simulink model "task3"  (R2023a)
settings: Solver=FixedStepAuto  StartTime=0.0  StopTime=10.0  RelTol=1e-3
libraries: simulink x9
settings Model: Creator=user  LastModifiedBy=user
settings OptimizationCC: DefaultParameterBehavior=Inlined  UseDivisionForNetSlopeComputation=on  GainParamInheritBuiltInType=on  UseFloatMulNetSlope=on  InlineInvariantSignals=on  PassReuseOutputArgsAs=Individual arguments  ZeroExternalMemoryAtStartup=off  ZeroInternalMemoryAtStartup=off  NoFixptDivByZeroProtection=on  EfficientFloat2IntCast=on  LifeSpan=1  OptimizeBlockOrder=speed  DifferentSizesBufferReuse=on  EfficientTunableParamExpr=on
settings DebuggingCC: ParameterTunabilityLossMsg=error
settings HardwareCC: ProdLongLongMode=on
settings SFSimCC: MATLABDynamicMemAlloc=off
settings RTWCC: Description=Embedded Coder  SystemTargetFile=ert.tlc  TemplateMakefile=ert_default_tmf
settings CodeAppCC: ForceParamTrailComments=on  IgnoreCustomStorageClasses=off  OperatorAnnotations=on  SimulinkDataObjDesc=on  SFDataObjDesc=on  CustomSymbolStrGlobalVar=rt$N$M  CustomSymbolStrType=$N$M  CustomSymbolStrFcn=$N$M$F  CustomSymbolStrMacro=$N$M  InsertBlockDesc=on
settings ERTTargetCC: TargetLangStandard=C99 (ISO)  GenerateSampleERTMain=on  IncludeMdlTerminateFcn=off  CombineSignalStateStructs=on  SupportComplex=off  SupportContinuousTime=on  InlinedParameterPlacement=NonHierarchical  ERTCustomFileTemplate=example_file_process.tlc  ERTFilePackagingFormat=CompactWithDataFile

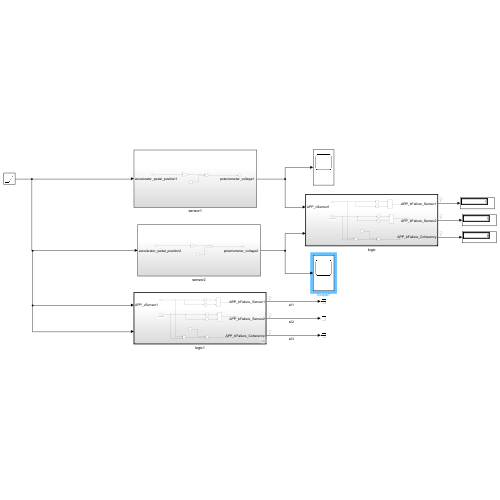
[thumbnail: Simulink's stored preview of the top-level diagram]
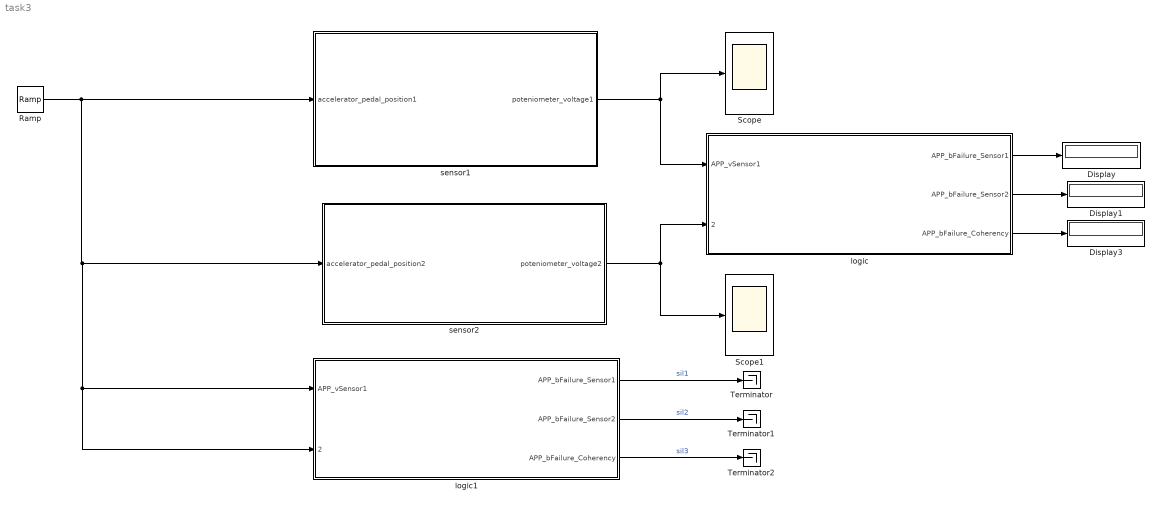
== system task3 ==
  Display : Display
  Display1 : Display
  Display3 : Display
  Ramp : simulink/Sources/Ramp  slope=1  start=0  InitialOutput=0
  Scope : Scope
  Scope1 : Scope
  Terminator : Terminator
  Terminator1 : Terminator
  Terminator2 : Terminator
  logic : Subsystem  TreatAsAtomicUnit=on
  logic1 : Subsystem  TreatAsAtomicUnit=on
  sensor1 : Subsystem
  sensor2 : Subsystem
  wires:
  sensor1/1("poteniometer_voltage1 ") -> Scope/1, logic/1("APP_vSensor1 ")
  sensor2/1("poteniometer_voltage2 ") -> logic/2(" "), Scope1/1
  logic/1(APP_bFailure_Sensor1) -> Display/1
  logic/2(APP_bFailure_Sensor2) -> Display1/1
  logic/3(APP_bFailure_Coherency) -> Display3/1
  Ramp/1 -> logic1/2(" "), logic1/1("APP_vSensor1 "), sensor2/1(accelerator_pedal_position2), sensor1/1("accelerator_pedal_position1 ")
  logic1/1(APP_bFailure_Sensor1) -> Terminator/1  "sil1"
  logic1/2(APP_bFailure_Sensor2) -> Terminator1/1  "sil2"
  logic1/3(APP_bFailure_Coherency) -> Terminator2/1  "sil3"

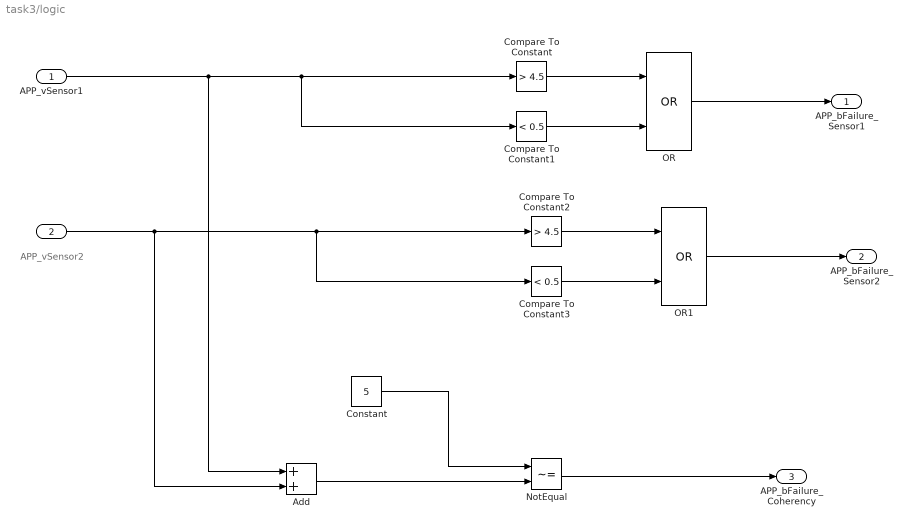
== system task3/logic ==
  note: APP_vSensor2
  "APP_vSensor1 " : Inport
  " " : Inport  Port=2
  Add : Sum
  Compare To Constant : simulink/Logic and Bit Operations/Compare To Constant  relop=>  const=4.5  OutDataTypeStr=boolean
  Compare To Constant1 : simulink/Logic and Bit Operations/Compare To Constant  relop=<  const=0.5  OutDataTypeStr=boolean
  Compare To Constant2 : simulink/Logic and Bit Operations/Compare To Constant  relop=>  const=4.5  OutDataTypeStr=boolean
  Compare To Constant3 : simulink/Logic and Bit Operations/Compare To Constant  relop=<  const=0.5  OutDataTypeStr=boolean
  Constant : Constant  Value=5
  NotEqual : RelationalOperator  Operator=~=  OutDataTypeStr=boolean  RndMeth=Simplest  InputSameDT=off
  OR : Logic  Operator=OR  AllPortsSameDT=off  OutDataTypeStr=boolean
  OR1 : Logic  Operator=OR  AllPortsSameDT=off  OutDataTypeStr=boolean
  APP_bFailure_Sensor1 : Outport
  APP_bFailure_Sensor2 : Outport  Port=2
  APP_bFailure_Coherency : Outport  Port=3
  wires:
  OR/1 -> APP_bFailure_Sensor1/1
  Compare To Constant/1 -> OR/1
  Compare To Constant1/1 -> OR/2
  "APP_vSensor1 "/1 -> Add/1, Compare To Constant1/1, Compare To Constant/1
  " "/1 -> Add/2, Compare To Constant2/1, Compare To Constant3/1
  Compare To Constant3/1 -> OR1/2
  Compare To Constant2/1 -> OR1/1
  OR1/1 -> APP_bFailure_Sensor2/1
  Constant/1 -> NotEqual/1
  Add/1 -> NotEqual/2
  NotEqual/1 -> APP_bFailure_Coherency/1

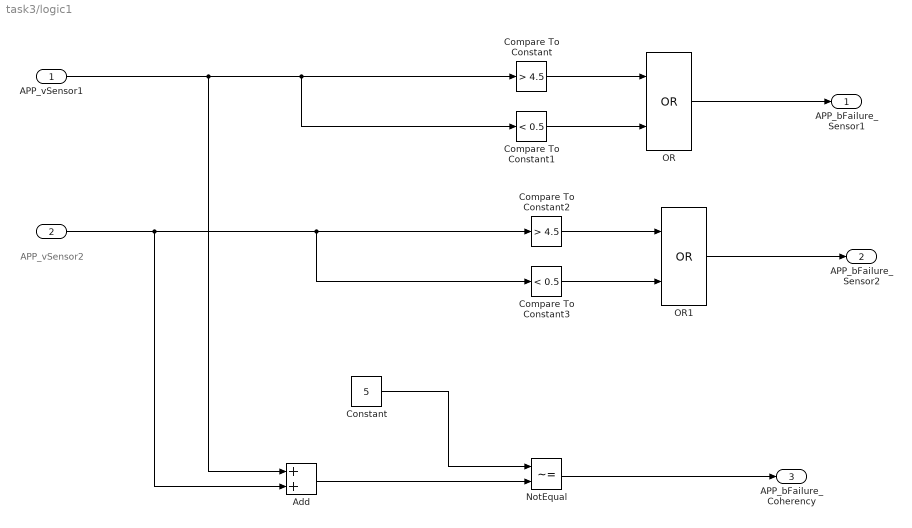
== system task3/logic1 ==
  note: APP_vSensor2
  "APP_vSensor1 " : Inport
  " " : Inport  Port=2
  Add : Sum
  Compare To Constant : simulink/Logic and Bit Operations/Compare To Constant  relop=>  const=4.5  OutDataTypeStr=boolean
  Compare To Constant1 : simulink/Logic and Bit Operations/Compare To Constant  relop=<  const=0.5  OutDataTypeStr=boolean
  Compare To Constant2 : simulink/Logic and Bit Operations/Compare To Constant  relop=>  const=4.5  OutDataTypeStr=boolean
  Compare To Constant3 : simulink/Logic and Bit Operations/Compare To Constant  relop=<  const=0.5  OutDataTypeStr=boolean
  Constant : Constant  Value=5
  NotEqual : RelationalOperator  Operator=~=  OutDataTypeStr=boolean  RndMeth=Simplest  InputSameDT=off
  OR : Logic  Operator=OR  AllPortsSameDT=off  OutDataTypeStr=boolean
  OR1 : Logic  Operator=OR  AllPortsSameDT=off  OutDataTypeStr=boolean
  APP_bFailure_Sensor1 : Outport
  APP_bFailure_Sensor2 : Outport  Port=2
  APP_bFailure_Coherency : Outport  Port=3
  wires:
  NotEqual/1 -> APP_bFailure_Coherency/1
  Add/1 -> NotEqual/2
  Constant/1 -> NotEqual/1
  OR1/1 -> APP_bFailure_Sensor2/1
  Compare To Constant2/1 -> OR1/1
  Compare To Constant3/1 -> OR1/2
  " "/1 -> Compare To Constant3/1, Compare To Constant2/1, Add/2
  "APP_vSensor1 "/1 -> Compare To Constant/1, Compare To Constant1/1, Add/1
  Compare To Constant1/1 -> OR/2
  Compare To Constant/1 -> OR/1
  OR/1 -> APP_bFailure_Sensor1/1

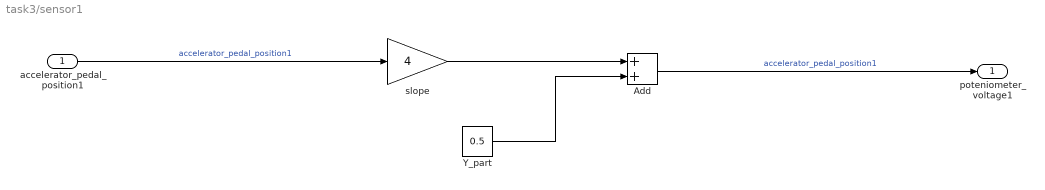
== system task3/sensor1 ==
  "accelerator_pedal_position1 " : Inport
  Add : Sum
  Y_part : Constant  Value=0.5
  slope : Gain  Gain=4
  "poteniometer_voltage1 " : Outport
  wires:
  Add/1 -> "poteniometer_voltage1 "/1  "accelerator_pedal_position1"
  "accelerator_pedal_position1 "/1 -> slope/1  "accelerator_pedal_position1"
  slope/1 -> Add/1
  Y_part/1 -> Add/2

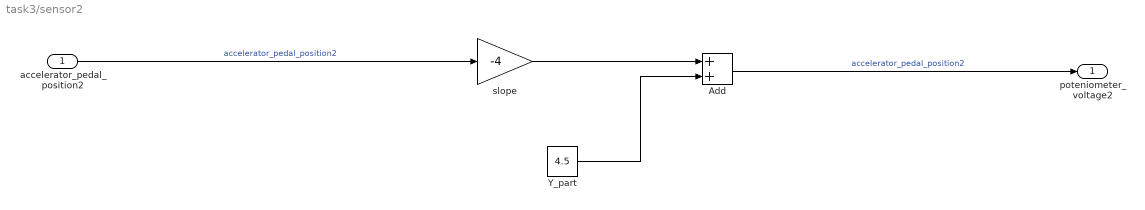
== system task3/sensor2 ==
  accelerator_pedal_position2 : Inport
  Add : Sum
  Y_part : Constant  Value=4.5
  slope : Gain  Gain=-4
  "poteniometer_voltage2 " : Outport
  wires:
  slope/1 -> Add/1
  Y_part/1 -> Add/2
  Add/1 -> "poteniometer_voltage2 "/1  "accelerator_pedal_position2"
  accelerator_pedal_position2/1 -> slope/1  "accelerator_pedal_position2"
